simulink model "second_CKT"  (R2025a)
settings: Solver=VariableStepAuto  StartTime=0.0  StopTime=0.1  RelTol=1e-3
values from neighbouring files (symbols this model uses):
  acf = 50    [seconddataentryckt.mat]
  acv = 10    [seconddataentryckt.mat]
  c = 0.0001    [seconddataentryckt.mat]
  l = 0.001    [seconddataentryckt.mat]
  r = 10    [seconddataentryckt.mat]
libraries: spsVoltageMeasurementLib x4, spsSeriesRLCBranchLib x3, spsACVoltageSourceLib x1, spsCurrentMeasurementLib x1, spspowerguiLib x1

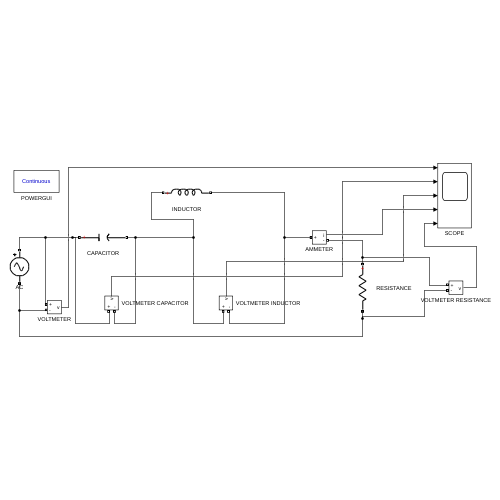
[thumbnail: Simulink's stored preview of the top-level diagram]
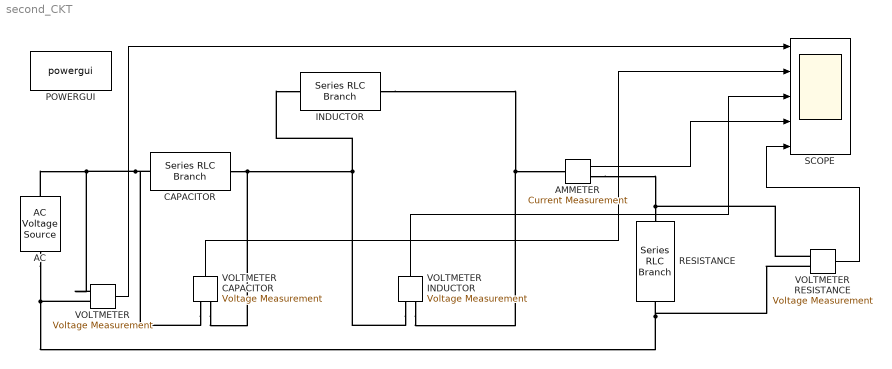
== system second_CKT ==
  AC : spsACVoltageSourceLib/AC Voltage Source  Amplitude=acv  Phase=0  Frequency=acf  SampleTime=0  Measurements=None  BusType=swing  Pref=10e3  Qref=0  Qmin=-inf  Qmax=+inf
  AMMETER : spsCurrentMeasurementLib/Current Measurement  PhasorSimulation=off  OutputType=Complex  PSBequivalent=0
  CAPACITOR : spsSeriesRLCBranchLib/Series RLC Branch  LConnTagsString=__new0  RConnTagsString=__new0  BranchType=C  Resistance=1  Inductance=1e-3  SetiL0=off  InitialCurrent=0  Capacitance=c  Setx0=off  InitialVoltage=0  Measurements=None
  INDUCTOR : spsSeriesRLCBranchLib/Series RLC Branch  LConnTagsString=__new0  RConnTagsString=__new0  BranchType=L  Resistance=1  Inductance=l  SetiL0=off  InitialCurrent=0  Capacitance=1e-6  Setx0=off  InitialVoltage=0  Measurements=None
  POWERGUI : spspowerguiLib/powergui  Priority=1  SimulationMode=Continuous  SampleTime=50e-6  frequency=60  Iterations=50  frequencyindice=50  Pbase=100e6  ErrMax=1e-4  UnitsV=kV  UnitsW=MW  buscounter=0  FunctionMessages=off  echomessages=off  EnableUseOfTLC=off  CurrentSourceSwitches=off  DisableSnubberDevices=off  DisableRonSwitches=off  DisableVfSwitches=off  DisplayEquations=off  AutomaticDiscreteSolvers=off  SolverType=Tustin/Backward Euler (TBE)  Interpol=off  ExternalGateDelay=off  methode=off  Ts=100  x0status=blocks  SPID=on  SwTol=0  HookPort=off  NonlinearTolerance=1e-4  nMaxIteration=100  ContinueOnMaxIteration=off  RestoreLinks=warning  ResistiveCurrentMeasurement=off  Frange=[0:2:500]  Ylog=off  Xlog=on  ShowGrid=off  save=off  variable=ZData  structure=0  ZoomFFT=off  StartTime=0.0  cycles=1  DisplayStyle=1  fundamental=60  FreqAxis=off  MaxFrequency=1000  frequencyindicesteady=1  RmsSteady=1  display=off
  RESISTANCE : spsSeriesRLCBranchLib/Series RLC Branch  LConnTagsString=__new0  RConnTagsString=__new0  BranchType=R  Resistance=r  Inductance=1e-3  SetiL0=off  InitialCurrent=0  Capacitance=1e-6  Setx0=off  InitialVoltage=0  Measurements=None
  SCOPE : Scope  NumInputPorts=5
      settings: ActiveDisplayYMinimum=-12.49989  ActiveDisplayYMaximum=12.49991
  VOLTMETER : spsVoltageMeasurementLib/Voltage Measurement  PhasorSimulation=off  OutputType=Complex  PSBequivalent=0
  VOLTMETER CAPACITOR : spsVoltageMeasurementLib/Voltage Measurement  PhasorSimulation=off  OutputType=Complex  PSBequivalent=0
  VOLTMETER INDUCTOR : spsVoltageMeasurementLib/Voltage Measurement  PhasorSimulation=off  OutputType=Complex  PSBequivalent=0
  VOLTMETER RESISTANCE : spsVoltageMeasurementLib/Voltage Measurement  PhasorSimulation=off  OutputType=Complex  PSBequivalent=0
  wires:
  VOLTMETER/1 -> SCOPE/1
  AMMETER/1 -> SCOPE/4
  VOLTMETER RESISTANCE/1 -> SCOPE/5
  VOLTMETER CAPACITOR/1 -> SCOPE/2
  VOLTMETER INDUCTOR/1 -> SCOPE/3
  connections:
  AC/RConn1 -- VOLTMETER CAPACITOR/LConn1 -- CAPACITOR/LConn1 -- VOLTMETER/LConn1
  CAPACITOR/RConn1 -- VOLTMETER CAPACITOR/LConn2 -- VOLTMETER INDUCTOR/LConn1 -- INDUCTOR/LConn1
  INDUCTOR/RConn1 -- AMMETER/LConn1 -- VOLTMETER INDUCTOR/LConn2
  AC/LConn1 -- VOLTMETER RESISTANCE/LConn2 -- RESISTANCE/RConn1 -- VOLTMETER/LConn2
  AMMETER/RConn1 -- VOLTMETER RESISTANCE/LConn1 -- RESISTANCE/LConn1
